simulink subsystem "EPS_Software"  (R2024a)
settings: Solver=VariableStepAuto  StartTime=0.0  StopTime=10.0  RelTol=1e-3
settings Model: Creator=dani  LastModifiedBy=dani

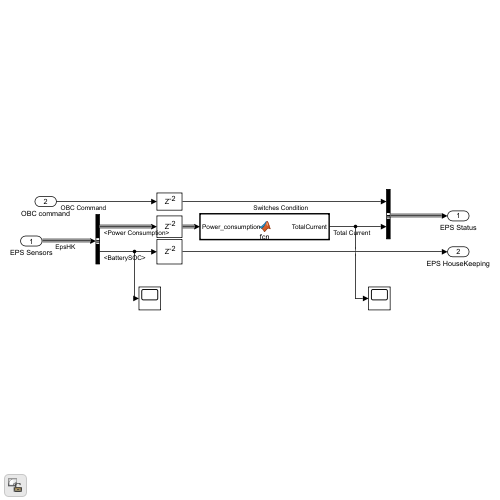
[thumbnail: Simulink's stored preview of the top-level diagram]
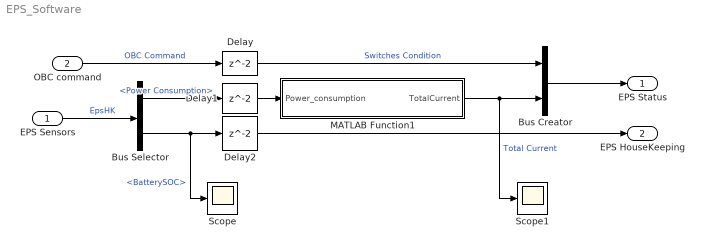
== system EPS_Software ==
  EPS Sensors : Inport
  OBC command : Inport  Port=2
  Bus Creator : BusCreator  Inputs=2
  Bus Selector : BusSelector  OutputSignals=Power Consumption,EPS HouseKeeping.BatterySOC
  Delay : Delay
  Delay1 : Delay
  Delay2 : Delay
  MATLAB Function1 : MATLAB Function  TreatAsAtomicUnit=on
  Scope : Scope
  Scope1 : Scope
  EPS Status : Outport
  EPS HouseKeeping : Outport  Port=2
  wires:
  EPS Sensors/1 -> Bus Selector/1  "EpsHK"
  Bus Creator/1 -> EPS Status/1
  OBC command/1 -> Delay/1  "OBC Command"
  MATLAB Function1/1(TotalCurrent) -> Bus Creator/2, Scope1/1  "Total Current"
  Bus Selector/1 -> Delay1/1  "<Power Consumption>"
  Bus Selector/2 -> Delay2/1, Scope/1  "<BatterySOC>"
  Delay/1 -> Bus Creator/1  "Switches Condition"
  Delay1/1 -> MATLAB Function1/1(Power_consumption)
  Delay2/1 -> EPS HouseKeeping/1

== matlab function EPS_Software/MATLAB Function1 ==
  data: Power_consumption input; TotalCurrent output
function TotalCurrent = fcn(Power_consumption)

TotalCurrent = 0;

for i = 1:length(Power_consumption)/2

    TotalCurrent = TotalCurrent + Power_consumption(2*(i)-1 ,1);
end
% TotalCurrent = sum(Power_consumption(:,2));

end
